simulink model "Problem6"  (R2020a)
settings: Solver=VariableStepAuto  StartTime=0.0  StopTime=10.0  RelTol=1e-3
settings Model: Creator=Shreyas  LastModifiedBy=Shreyas

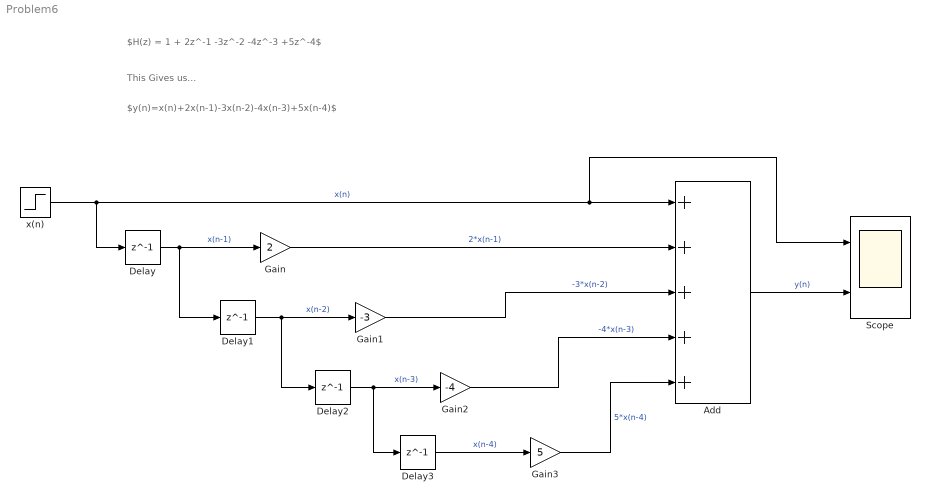
== system Problem6 ==
  note: $y(n)=x(n)+2x(n-1)-3x(n-2)-4x(n-3)+5x(n-4)$
  note: This Gives us...
  note: $H(z) = 1 + 2z^-1 -3z^-2 -4z^-3 +5z^-4$
  Add : Sum  Inputs=+++++
  Delay{,1..3} (4 alike) : Delay  DelayLength=1
  Gain : Gain  Gain=2
  Gain1 : Gain  Gain=-3
  Gain2 : Gain  Gain=-4
  Gain3 : Gain  Gain=5
  Scope : Scope  NumInputPorts=2
  x(n) : Step  SampleTime=0
  wires:
  Delay/1 -> Delay1/1, Gain/1  "x(n-1)"
  Delay1/1 -> Delay2/1, Gain1/1  "x(n-2)"
  Delay2/1 -> Delay3/1, Gain2/1  "x(n-3)"
  Delay3/1 -> Gain3/1  "x(n-4)"
  x(n)/1 -> Delay/1, Scope/1, Add/1  "x(n)"
  Gain3/1 -> Add/5  "5*x(n-4)"
  Gain2/1 -> Add/4  "-4*x(n-3)"
  Gain1/1 -> Add/3  "-3*x(n-2)"
  Gain/1 -> Add/2  "2*x(n-1)"
  Add/1 -> Scope/2  "y(n)"
